simulink model "HumanoidModel_ResidualRL"  (R2025b)
settings: Solver=daessc  StartTime=0.0  StopTime=11  RelTol=1e-3  AbsTol=1e-3
PreLoadFcn:
  | addpath(fullfile('ImportedURDFSupport','Geometries'));
  | addpath(fullfile('ImportedURDFSupport','Data'));
undefined symbols (not defined in the file): kd_ankle_vy, kd_ankle_wx, kd_hip_sag_vx, kd_hip_sag_wy, kd_hip_vy, kd_hip_vz, kd_hip_wx, kp_ankle_qx, kp_ankle_y, kp_hip_dz, kp_hip_qx, kp_hip_sag_qy, kp_hip_sag_x, kp_hip_y, params, residualRLActionPenaltyWeight, residualRLActionRatePenaltyWeight, residualRLAliveReward, residualRLChannelMap, residualRLEnabled, residualRLLeftFootLoadMap, residualRLManualAction, residualRLNominalFootLoad_N, residualRLObservationInverseScales, residualRLRewardStateWeights, residualRLRightFootLoadMap, residualRLSampleTime_s, residualRLTerminalPenalty, residualRLTorqueLimit_Nm, residualRLUseAgent, robustnessForceDuration_s, robustnessForceStart_s, robustnessForceVector_N, Rx_ref, u_ankle_pitch, u_hip_frontal, u_hip_sagittal, u_knee, u_shoulder_frontal, X, Y, y_ref, Z
libraries: sm_lib x155, nesl_utility x96, simulink_extras x18, simulink x5, robotmaniplib x1, rllib x1
(part 2 of 6)

== system HumanoidModel_ResidualRL/Torque Reordering1 ==
  In1 : Inport
  Bus Creator3 : BusCreator  Inputs=12
  Demux : Demux  Outputs=22
  Gain{1..12} (12 alike) : Gain
  Scope5 : Scope
      settings: ActiveDisplayYMinimum=-30.863133772002811  ActiveDisplayYMaximum=8.6957298127878211  DataLoggingVariableName=ScopeData5
  Out1 : Outport
  wires:
  In1/1 -> Demux/1
  Bus Creator3/1 -> Scope5/1, Out1/1
  Demux/12 -> Gain12/1  "right_hip_frontal"
  Demux/14 -> Gain6/1  "right_knee"
  Demux/16 -> Gain11/1  "right_ankle_pitch"
  Demux/13 -> Gain8/1  "right_hip_sagittal"
  Demux/11 -> Gain7/1  "right_hip_transverse"
  Demux/15 -> Gain10/1  "right_ankle_roll"
  Demux/18 -> Gain4/1  "left_hip_frontal"
  Gain4/1 -> Bus Creator3/7  "left_hip_frontal"
  Demux/20 -> Gain1/1  "left_knee"
  Gain1/1 -> Bus Creator3/8  "left_knee"
  Demux/22 -> Gain9/1  "left_ankle_pitch"
  Demux/19 -> Gain2/1  "left_hip_sagittal"
  Gain2/1 -> Bus Creator3/10  "left_hip_sagittal"
  Demux/17 -> Gain3/1  "left_hip_transverse"
  Gain3/1 -> Bus Creator3/11  "left_hip_transverse"
  Demux/21 -> Gain5/1  "left_ankle_roll"
  Gain5/1 -> Bus Creator3/12  "left_ankle_roll"
  Gain6/1 -> Bus Creator3/2  "right_knee"
  Gain7/1 -> Bus Creator3/5  "right_hip_transverse"
  Gain8/1 -> Bus Creator3/4  "right_hip_sagittal"
  Gain9/1 -> Bus Creator3/9  "left_ankle_pitch"
  Gain10/1 -> Bus Creator3/6  "right_ankle_roll"
  Gain11/1 -> Bus Creator3/3  "right_ankle_pitch"
  Gain12/1 -> Bus Creator3/1  "right_hip_frontal"

== system HumanoidModel_ResidualRL/Control Input/Left ankle feedback ==
  qx : Inport
  wx : Inport  Port=2
  vy : Inport  Port=3
  y : Inport  Port=4
  Constant2 : Constant  Value=u_ankle_pitch
  Gain : Gain  Gain=kd_ankle_wx
  Gain1 : Gain  Gain=kp_ankle_qx
  Gain2 : Gain  Gain=kp_ankle_y
  Gain3 : Gain  Gain=kd_ankle_vy
  Subtract : Sum  Inputs=+-
  Subtract1 : Sum  Inputs=+-
  Sum : Sum  Inputs=|++++
  Sum1 : Sum  Inputs=|++
  qx_ref : Constant  Value=Rx_ref
  y_ref : Constant  Value=y_ref
  Out1 : Outport
  wires:
  Sum/1 -> Out1/1
  Subtract/1 -> Gain1/1
  Gain1/1 -> Sum/1
  Gain/1 -> Sum/2
  wx/1 -> Gain/1
  qx/1 -> Subtract/1
  qx_ref/1 -> Subtract/2
  Sum1/1 -> Sum/4
  Gain3/1 -> Sum1/2
  y_ref/1 -> Subtract1/2
  Gain2/1 -> Sum1/1
  Subtract1/1 -> Gain2/1
  y/1 -> Subtract1/1
  vy/1 -> Gain3/1
  Constant2/1 -> Sum/3

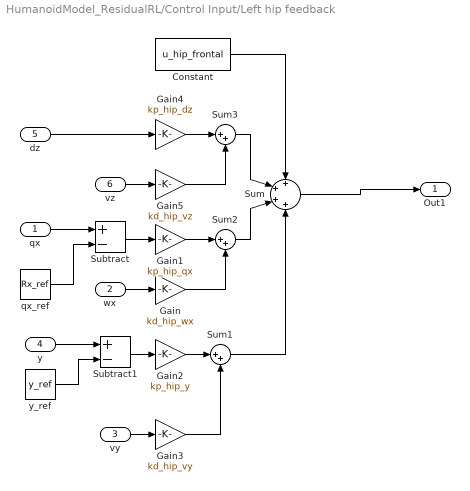
== system HumanoidModel_ResidualRL/Control Input/Left hip feedback ==
  qx : Inport
  wx : Inport  Port=2
  vy : Inport  Port=3
  y : Inport  Port=4
  dz : Inport  Port=5
  vz : Inport  Port=6
  Constant : Constant  Value=u_hip_frontal
  Gain : Gain  Gain=kd_hip_wx
  Gain1 : Gain  Gain=kp_hip_qx
  Gain2 : Gain  Gain=kp_hip_y
  Gain3 : Gain  Gain=kd_hip_vy
  Gain4 : Gain  Gain=kp_hip_dz
  Gain5 : Gain  Gain=kd_hip_vz
  Subtract : Sum  Inputs=+-
  Subtract1 : Sum  Inputs=+-
  Sum : Sum  Inputs=++++
  Sum1 : Sum  Inputs=|++
  Sum2 : Sum  Inputs=|++
  Sum3 : Sum  Inputs=|++
  qx_ref : Constant  Value=Rx_ref
  y_ref : Constant  Value=y_ref
  Out1 : Outport
  wires:
  Gain1/1 -> Sum2/1
  Gain4/1 -> Sum3/1
  Sum3/1 -> Sum/2
  vz/1 -> Gain5/1
  Gain2/1 -> Sum1/1
  Gain/1 -> Sum2/2
  Subtract1/1 -> Gain2/1
  Sum1/1 -> Sum/4
  Subtract/1 -> Gain1/1
  wx/1 -> Gain/1
  Gain3/1 -> Sum1/2
  y/1 -> Subtract1/1
  vy/1 -> Gain3/1
  qx/1 -> Subtract/1
  y_ref/1 -> Subtract1/2
  Sum/1 -> Out1/1
  Gain5/1 -> Sum3/2
  Sum2/1 -> Sum/3
  qx_ref/1 -> Subtract/2
  dz/1 -> Gain4/1
  Constant/1 -> Sum/1

== system HumanoidModel_ResidualRL/Control Input/Left hip sagittal feedback ==
  qy : Inport
  wy : Inport  Port=2
  x : Inport  Port=3
  vx : Inport  Port=4
  Gain : Gain  Gain=kp_hip_sag_qy
  Gain1 : Gain  Gain=kd_hip_sag_wy
  Gain2 : Gain  Gain=kd_hip_sag_vx
  Gain3 : Gain  Gain=kp_hip_sag_x
  Nominal hip sagittal u : Constant  Value=u_hip_sagittal
  Sum : Sum  Inputs=+++++
  Out1 : Outport
  wires:
  Sum/1 -> Out1/1
  vx/1 -> Gain2/1
  x/1 -> Gain3/1
  Gain2/1 -> Sum/4
  Gain3/1 -> Sum/3
  Gain1/1 -> Sum/2
  Gain/1 -> Sum/1
  wy/1 -> Gain1/1
  qy/1 -> Gain/1
  Nominal hip sagittal u/1 -> Sum/5

== system HumanoidModel_ResidualRL/Control Input/Right ankle feedback ==
  qx : Inport
  wx : Inport  Port=2
  vy : Inport  Port=3
  y : Inport  Port=4
  Constant2 : Constant  Value=u_ankle_pitch
  Gain : Gain  Gain=kd_ankle_wx
  Gain1 : Gain  Gain=kp_ankle_qx
  Gain2 : Gain  Gain=kp_ankle_y
  Gain3 : Gain  Gain=kd_ankle_vy
  Subtract : Sum  Inputs=+-
  Subtract1 : Sum  Inputs=+-
  Sum : Sum  Inputs=|++++
  Sum1 : Sum  Inputs=|++
  qx_ref : Constant  Value=Rx_ref
  y_ref : Constant  Value=y_ref
  Out1 : Outport
  wires:
  wx/1 -> Gain/1
  Gain/1 -> Sum/2
  Gain1/1 -> Sum/1
  Sum/1 -> Out1/1
  Subtract/1 -> Gain1/1
  qx/1 -> Subtract/1
  qx_ref/1 -> Subtract/2
  Sum1/1 -> Sum/4
  Gain3/1 -> Sum1/2
  y_ref/1 -> Subtract1/2
  Gain2/1 -> Sum1/1
  Subtract1/1 -> Gain2/1
  y/1 -> Subtract1/1
  vy/1 -> Gain3/1
  Constant2/1 -> Sum/3

== system HumanoidModel_ResidualRL/Control Input/Right hip feedback ==
  qx : Inport
  wx : Inport  Port=2
  vy : Inport  Port=3
  y : Inport  Port=4
  dz : Inport  Port=5
  vz : Inport  Port=6
  Constant : Constant  Value=u_hip_frontal
  Gain : Gain  Gain=kd_hip_wx
  Gain1 : Gain  Gain=kp_hip_qx
  Gain2 : Gain  Gain=kp_hip_y
  Gain3 : Gain  Gain=kd_hip_vy
  Gain4 : Gain  Gain=kp_hip_dz
  Gain5 : Gain  Gain=kd_hip_vz
  Subtract : Sum  Inputs=+-
  Subtract1 : Sum  Inputs=+-
  Sum : Sum  Inputs=++++
  Sum1 : Sum  Inputs=|++
  Sum2 : Sum  Inputs=|++
  Sum3 : Sum  Inputs=|++
  qx_ref : Constant  Value=Rx_ref
  y_ref : Constant  Value=y_ref
  Out1 : Outport
  wires:
  qx_ref/1 -> Subtract/2
  qx/1 -> Subtract/1
  Subtract/1 -> Gain1/1
  Sum/1 -> Out1/1
  wx/1 -> Gain/1
  y/1 -> Subtract1/1
  y_ref/1 -> Subtract1/2
  Subtract1/1 -> Gain2/1
  Gain2/1 -> Sum1/1
  vy/1 -> Gain3/1
  Gain3/1 -> Sum1/2
  Sum1/1 -> Sum/4
  Gain1/1 -> Sum2/1
  Gain/1 -> Sum2/2
  Sum2/1 -> Sum/3
  dz/1 -> Gain4/1
  vz/1 -> Gain5/1
  Gain4/1 -> Sum3/1
  Gain5/1 -> Sum3/2
  Sum3/1 -> Sum/2
  Constant/1 -> Sum/1  "Right Hip Frontal"

== system HumanoidModel_ResidualRL/Control Input/Right hip sagittal feedback ==
  qy : Inport
  wy : Inport  Port=2
  x : Inport  Port=3
  vx : Inport  Port=4
  Gain : Gain  Gain=kp_hip_sag_qy
  Gain1 : Gain  Gain=kd_hip_sag_wy
  Gain2 : Gain  Gain=kd_hip_sag_vx
  Gain3 : Gain  Gain=kp_hip_sag_x
  Nominal hip sagittal u : Constant  Value=u_hip_sagittal
  Sum : Sum  Inputs=+++++
  Out1 : Outport
  wires:
  qy/1 -> Gain/1
  wy/1 -> Gain1/1
  Gain/1 -> Sum/1
  Gain1/1 -> Sum/2
  Gain3/1 -> Sum/3
  Gain2/1 -> Sum/4
  x/1 -> Gain3/1
  vx/1 -> Gain2/1
  Sum/1 -> Out1/1
  Nominal hip sagittal u/1 -> Sum/5

== system HumanoidModel_ResidualRL/Humanoid Robot/Arms ==
  Torque Input : Inport
  Bus Creator : BusCreator  Inputs=2
  Demux : Demux  Outputs=2
  Left Arm : Subsystem
  Right Arm : Subsystem
  Right Shoulder : PMIOPort  Side=Left
  Left Shoulder : PMIOPort  Port=2  Side=Left
  Arms Joint Sensing : Outport
  wires:
  Torque Input/1 -> Demux/1
  Demux/1 -> Right Arm/1(Torque Input)
  Demux/2 -> Left Arm/1(Torque Input)
  Bus Creator/1 -> Arms Joint Sensing/1
  Left Arm/1(Sensing) -> Bus Creator/2
  Right Arm/1(Sensing) -> Bus Creator/1
  connections:
  Left Arm/LConn1 -- Left Shoulder/RConn1
  Right Arm/LConn1 -- Right Shoulder/RConn1

== system HumanoidModel_ResidualRL/Humanoid Robot/Foot Contact Modelling ==
  Bus Creator : BusCreator  Inputs=2
  Bus Creator1 : BusCreator  Inputs=2
  Left Foot Contact : Subsystem  AncestorBlock=sm_humanoid_walker_lib/Humanoid Robot/Foot Contact Modelling/Right Foot Contact
  Right Foot Contact : Subsystem
  Right Foot Contact Points : PMIOPort  Side=Left
  Left Foot Contact Points : PMIOPort  Port=2  Side=Left
  Feet Contact : PMIOPort  Port=3  Side=Left
  Total Contact Sensing : Outport
  Contact Sensing : Outport  Port=2
  wires:
  Bus Creator/1 -> Total Contact Sensing/1
  Right Foot Contact/1(Foot Force) -> Bus Creator/1  "rightContactTotal"
  Left Foot Contact/1(Foot Force) -> Bus Creator/2  "leftContactTotal"
  Bus Creator1/1 -> Contact Sensing/1
  Right Foot Contact/2(Contact Point Forces) -> Bus Creator1/1  "rightContact"
  Left Foot Contact/2(Contact Point Forces) -> Bus Creator1/2  "leftContact"
  connections:
  Left Foot Contact/LConn1 -- Left Foot Contact Points/RConn1
  Feet Contact/RConn1 -- Left Foot Contact/RConn1 -- Right Foot Contact/RConn1
  Right Foot Contact/LConn1 -- Right Foot Contact Points/RConn1

== system HumanoidModel_ResidualRL/Humanoid Robot/Legs ==
  Torque Input : Inport
  Bus Creator : BusCreator  Inputs=2
  Demux : Demux  Outputs=2
  Left Leg : Subsystem
  Right leg : Subsystem
  Right Hip : PMIOPort  Side=Left
  Right Foot : PMIOPort  Port=2  Side=Right
  Left Foot : PMIOPort  Port=3  Side=Right
  Left Hip : PMIOPort  Port=4  Side=Left
  Joint Sensing : Outport
  wires:
  Demux/2 -> Left Leg/1(Torque Input)
  Left Leg/1(Sensing) -> Bus Creator/2
  Torque Input/1 -> Demux/1
  Demux/1 -> Right leg/1(Torque Input)
  Bus Creator/1 -> Joint Sensing/1
  Right leg/1(Sensing) -> Bus Creator/1
  connections:
  Right Hip/RConn1 -- Right leg/LConn1
  Left Foot/RConn1 -- Left Leg/RConn1
  Right Foot/RConn1 -- Right leg/RConn1
  Left Hip/RConn1 -- Left Leg/LConn1

== system HumanoidModel_ResidualRL/Humanoid Robot/Torso and Head ==
  Cover : sm_lib/Body Elements/File Solid  ExtGeomFileName=sm_humanoid_walker_cover.stp  UnitType=FromFile  ExtGeomFileUnits=m  StepReaderType=HEX  ExportConvexHullGeometry=off  InertiaType=CalculateFromGeometry  BasedOnType=Density  Density=headDensity  DensityUnits=kg/m^3  Mass=0  MassUnits=kg  CenterOfMass=[0, 0, 0]  CenterOfMassUnits=m  MomentsOfInertia=[0, 0, 0]  MomentsOfInertiaUnits=kg*m^2  ProductsOfInertia=[0, 0, 0]  ProductsOfInertiaUnits=kg*m^2  GraphicType=FromGeometry  MarkerShape=Sphere  MarkerSize=10  GraphicVisPropType=SimpleVisualProperties  GraphicDiffuseColor=[1, 1, 1]  GraphicOpacity=1  GraphicSpecularColor=[0.5 0.5 0.5 1.0]  GraphicAmbientColor=[0.15 0.15 0.15 1.0]  GraphicEmissiveColor=[0.0 0.0 0.0 1.0]  GraphicShininess=75  DoExposeReferenceFrame=on  SerializedFrames=<Frames/>
  Head : sm_lib/Body Elements/File Solid  ExtGeomFileName=sm_humanoid_walker_head.stp  UnitType=FromFile  ExtGeomFileUnits=m  StepReaderType=HEX  ExportConvexHullGeometry=off  InertiaType=CalculateFromGeometry  BasedOnType=Density  Density=headDensity  DensityUnits=kg/m^3  Mass=0  MassUnits=kg  CenterOfMass=[0, 0, 0]  CenterOfMassUnits=m  MomentsOfInertia=[0, 0, 0]  MomentsOfInertiaUnits=kg*m^2  ProductsOfInertia=[0, 0, 0]  ProductsOfInertiaUnits=kg*m^2  GraphicType=FromGeometry  MarkerShape=Sphere  MarkerSize=10  GraphicVisPropType=SimpleVisualProperties  GraphicDiffuseColor=[0.0 0.0 0.0]  GraphicOpacity=1  GraphicSpecularColor=[0.5 0.5 0.5 1.0]  GraphicAmbientColor=[0.15 0.15 0.15 1.0]  GraphicEmissiveColor=[0.0 0.0 0.0 1.0]  GraphicShininess=75  DoExposeReferenceFrame=on  SerializedFrames=<Frames/>
  Head Origin Transformation : sm_lib/Frames and Transforms/Rigid Transform  RotationMethod=RotationSequence  FollAlignAxisA=+X  BaseAlignAxisA=+Y  FollAlignAxisB=+Y  BaseAlignAxisB=+Z  RotationStandardAxis=+Z  RotationAngle=0.0  RotationAngleUnits=deg  RotationArbitraryAxis=[0 0 1]  RotationSequenceAxes=BaseAxes  RotationSequence=XYZ  RotationSequenceAngles=[0, 0, 0]  RotationSequenceAnglesUnits=rad  RotationMatrix=[1 0 0; 0 1 0; 0 0 1]  Quaternion=[1 0 0 0]  TranslationMethod=Cartesian  TranslationCartesianOffset=[0, 0, 0.06414]*3.5  TranslationCartesianOffsetUnits=m  TranslationStandardAxis=+Z  TranslationStandardOffset=0  TranslationStandardOffsetUnits=m  TranslationROffset=0  TranslationROffsetUnits=m  TranslationThetaOffset=0  TranslationThetaOffsetUnits=deg  TranslationZOffset=0  TranslationZOffsetUnits=m
  Neck : sm_lib/Body Elements/File Solid  ExtGeomFileName=sm_humanoid_walker_neck.stp  UnitType=FromFile  ExtGeomFileUnits=m  StepReaderType=HEX  ExportConvexHullGeometry=off  InertiaType=CalculateFromGeometry  BasedOnType=Density  Density=headDensity  DensityUnits=kg/m^3  Mass=0  MassUnits=kg  CenterOfMass=[0, 0, 0]  CenterOfMassUnits=m  MomentsOfInertia=[0, 0, 0]  MomentsOfInertiaUnits=kg*m^2  ProductsOfInertia=[0, 0, 0]  ProductsOfInertiaUnits=kg*m^2  GraphicType=FromGeometry  MarkerShape=Sphere  MarkerSize=10  GraphicVisPropType=SimpleVisualProperties  GraphicDiffuseColor=[0.0 0.0 0.0]  GraphicOpacity=1  GraphicSpecularColor=[0.5 0.5 0.5 1.0]  GraphicAmbientColor=[0.15 0.15 0.15 1.0]  GraphicEmissiveColor=[0.0 0.0 0.0 1.0]  GraphicShininess=75  DoExposeReferenceFrame=on  SerializedFrames=<Frames/>
  Neck Origin Tranformation : sm_lib/Frames and Transforms/Rigid Transform  RotationMethod=RotationSequence  FollAlignAxisA=+X  BaseAlignAxisA=+Y  FollAlignAxisB=+Y  BaseAlignAxisB=+Z  RotationStandardAxis=+Z  RotationAngle=0.0  RotationAngleUnits=deg  RotationArbitraryAxis=[0 0 1]  RotationSequenceAxes=BaseAxes  RotationSequence=XYZ  RotationSequenceAngles=[0, 0, 0]  RotationSequenceAnglesUnits=rad  RotationMatrix=[1 0 0; 0 1 0; 0 0 1]  Quaternion=[1 0 0 0]  TranslationMethod=Cartesian  TranslationCartesianOffset=[0, 0, 0.01016]*3.5  TranslationCartesianOffsetUnits=m  TranslationStandardAxis=+Z  TranslationStandardOffset=0  TranslationStandardOffsetUnits=m  TranslationROffset=0  TranslationROffsetUnits=m  TranslationThetaOffset=0  TranslationThetaOffsetUnits=deg  TranslationZOffset=0  TranslationZOffsetUnits=m
  Shoulder : sm_lib/Body Elements/File Solid  ExtGeomFileName=sm_humanoid_walker_shoulder.stp  UnitType=FromFile  ExtGeomFileUnits=m  StepReaderType=HEX  ExportConvexHullGeometry=off  InertiaType=CalculateFromGeometry  BasedOnType=Density  Density=shoulderDensity  DensityUnits=kg/m^3  Mass=0  MassUnits=kg  CenterOfMass=[0, 0, 0]  CenterOfMassUnits=m  MomentsOfInertia=[0, 0, 0]  MomentsOfInertiaUnits=kg*m^2  ProductsOfInertia=[0, 0, 0]  ProductsOfInertiaUnits=kg*m^2  GraphicType=FromGeometry  MarkerShape=Sphere  MarkerSize=10  GraphicVisPropType=SimpleVisualProperties  GraphicDiffuseColor=[1.0 0.6 0.6]  GraphicOpacity=1  GraphicSpecularColor=[0.5 0.5 0.5 1.0]  GraphicAmbientColor=[0.15 0.15 0.15 1.0]  GraphicEmissiveColor=[0.0 0.0 0.0 1.0]  GraphicShininess=75  DoExposeReferenceFrame=on  SerializedFrames=<Frames/>
  Shoulder Origin Transformation : sm_lib/Frames and Transforms/Rigid Transform  RotationMethod=RotationSequence  FollAlignAxisA=+X  BaseAlignAxisA=+Y  FollAlignAxisB=+Y  BaseAlignAxisB=+Z  RotationStandardAxis=+Z  RotationAngle=0.0  RotationAngleUnits=deg  RotationArbitraryAxis=[0 0 1]  RotationSequenceAxes=BaseAxes  RotationSequence=XYZ  RotationSequenceAngles=[0, 0, 0]  RotationSequenceAnglesUnits=rad  RotationMatrix=[1 0 0; 0 1 0; 0 0 1]  Quaternion=[1 0 0 0]  TranslationMethod=Cartesian  TranslationCartesianOffset=[0, 0, -0.0399]*3.5  TranslationCartesianOffsetUnits=m  TranslationStandardAxis=+Z  TranslationStandardOffset=0  TranslationStandardOffsetUnits=m  TranslationROffset=0  TranslationROffsetUnits=m  TranslationThetaOffset=0  TranslationThetaOffsetUnits=deg  TranslationZOffset=0  TranslationZOffsetUnits=m
  Trunk : sm_lib/Body Elements/File Solid  ExtGeomFileName=sm_humanoid_walker_trunk.stp  UnitType=FromFile  ExtGeomFileUnits=km  StepReaderType=HEX  ExportConvexHullGeometry=off  InertiaType=CalculateFromGeometry  BasedOnType=Density  Density=trunkDensity  DensityUnits=kg/m^3  Mass=0  MassUnits=kg  CenterOfMass=[0, 0, 0]  CenterOfMassUnits=m  MomentsOfInertia=[0, 0, 0]  MomentsOfInertiaUnits=kg*m^2  ProductsOfInertia=[0, 0, 0]  ProductsOfInertiaUnits=kg*m^2  GraphicType=FromGeometry  MarkerShape=Sphere  MarkerSize=10  GraphicVisPropType=SimpleVisualProperties  GraphicDiffuseColor=[1.0 0.2 0.2]  GraphicOpacity=1  GraphicSpecularColor=[0.5 0.5 0.5 1.0]  GraphicAmbientColor=[0.15 0.15 0.15 1.0]  GraphicEmissiveColor=[0.0 0.0 0.0 1.0]  GraphicShininess=75  DoExposeReferenceFrame=on  SerializedFrames=<Frames/>
  Torso : PMIOPort  Side=Left
  Torso Ref : PMIOPort  Port=2  Side=Right
  connections:
  Neck/RConn1 -- Head Origin Transformation/LConn1 -- Neck Origin Tranformation/RConn1
  Neck Origin Tranformation/LConn1 -- Shoulder Origin Transformation/RConn1 -- Shoulder/RConn1
  Cover/RConn1 -- Head Origin Transformation/RConn1 -- Head/RConn1
  Trunk/RConn1 -- Torso/RConn1 -- Torso Ref/RConn1 -- Shoulder Origin Transformation/LConn1

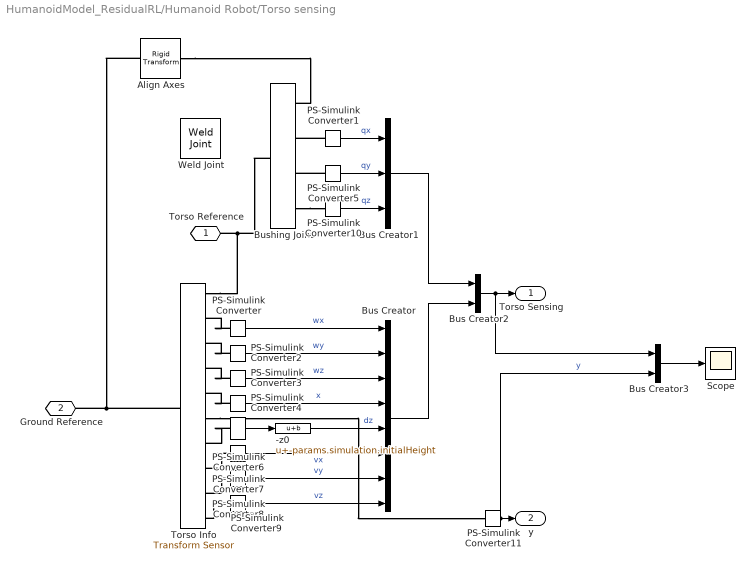
== system HumanoidModel_ResidualRL/Humanoid Robot/Torso sensing ==
  -z0 : Bias  Bias=-params.simulation.initialHeight  SaturateOnIntegerOverflow=off
  Align Axes : sm_lib/Frames and Transforms/Rigid Transform  RotationMethod=StandardAxis  FollAlignAxisA=+X  BaseAlignAxisA=+Y  FollAlignAxisB=+Y  BaseAlignAxisB=+Z  RotationStandardAxis=+Z  RotationAngle=180  RotationAngleUnits=deg  RotationArbitraryAxis=[0 0 1]  RotationSequenceAxes=FollowerAxes  RotationSequence=XYX  RotationSequenceAngles=[0 0 0]  RotationSequenceAnglesUnits=deg  RotationMatrix=[1 0 0; 0 1 0; 0 0 1]  Quaternion=[1 0 0 0]  TranslationMethod=None  TranslationCartesianOffset=[0 0 0]  TranslationCartesianOffsetUnits=m  TranslationStandardAxis=+Z  TranslationStandardOffset=0  TranslationStandardOffsetUnits=m  TranslationROffset=0  TranslationROffsetUnits=m  TranslationThetaOffset=0  TranslationThetaOffsetUnits=deg  TranslationZOffset=0  TranslationZOffsetUnits=m
  Bus Creator : BusCreator  Inputs=8
  Bus Creator1 : BusCreator  Inputs=3
  Bus Creator2 : BusCreator  Inputs=2
  Bus Creator3 : BusCreator  Inputs=2
  Bushing Joint : sm_lib/Joints/Bushing Joint  JointMode=Normal  CompositeWrenchDir=FollowerOnBase  CompositeWrenchFrame=BaseFrame  SenseConstraintForce=off  SenseConstraintTorque=off  SenseTotalForce=off  SenseTotalTorque=off  PxPositionTargetSpecify=off  PxPositionTargetPriority=High  PxPositionTargetValue=0  PxPositionTargetValueUnits=m  PxVelocityTargetSpecify=off  PxVelocityTargetPriority=High  PxVelocityTargetValue=0  PxVelocityTargetValueUnits=m/s  PxEquilibriumPosition=0  PxEquilibriumPositionUnits=m  PxSpringStiffness=0  PxSpringStiffnessUnits=N/m  PxDampingCoefficient=0  PxDampingCoefficientUnits=N/(m/s)  PxLowerLimitSpecify=off  PxLowerLimitBound=-0.02  PxLowerLimitBoundUnits=m  PxLowerLimitStiffness=1e6  PxLowerLimitStiffnessUnits=N/m  PxLowerLimitDamping=1e3  PxLowerLimitDampingUnits=N/(m/s)  PxLowerLimitTransitionRegionWidth=1e-4  PxLowerLimitTransitionRegionWidthUnits=m  PxUpperLimitSpecify=off  PxUpperLimitBound=0.02  PxUpperLimitBoundUnits=m  PxUpperLimitStiffness=1e6  PxUpperLimitStiffnessUnits=N/m  PxUpperLimitDamping=1e3  PxUpperLimitDampingUnits=N/(m/s)  PxUpperLimitTransitionRegionWidth=1e-4  PxUpperLimitTransitionRegionWidthUnits=m  PxTorqueActuationMode=NoTorque  PxMotionActuationMode=ComputedMotion  PxSensePosition=off  PxSenseVelocity=off  PxSenseAcceleration=off  PxSenseTorqueForce=off  PxSenseLowerLimitTorqueForce=off  PxSenseUpperLimitTorqueForce=off  PyPositionTargetSpecify=off  PyPositionTargetPriority=High  PyPositionTargetValue=0  PyPositionTargetValueUnits=m  PyVelocityTargetSpecify=off  PyVelocityTargetPriority=High  PyVelocityTargetValue=0  PyVelocityTargetValueUnits=m/s  PyEquilibriumPosition=0  PyEquilibriumPositionUnits=m  PySpringStiffness=0  PySpringStiffnessUnits=N/m  PyDampingCoefficient=0  PyDampingCoefficientUnits=N/(m/s)  PyLowerLimitSpecify=off  PyLowerLimitBound=-1  PyLowerLimitBoundUnits=m  PyLowerLimitStiffness=1e6  PyLowerLimitStiffnessUnits=N/m  PyLowerLimitDamping=1e3  PyLowerLimitDampingUnits=N/(m/s)  PyLowerLimitTransitionRegionWidth=1e-4  PyLowerLimitTransitionRegionWidthUnits=m  PyUpperLimitSpecify=off  PyUpperLimitBound=1  PyUpperLimitBoundUnits=m  PyUpperLimitStiffness=1e6  PyUpperLimitStiffnessUnits=N/m  PyUpperLimitDamping=1e3  PyUpperLimitDampingUnits=N/(m/s)  PyUpperLimitTransitionRegionWidth=1e-4  PyUpperLimitTransitionRegionWidthUnits=m  PyTorqueActuationMode=NoTorque  PyMotionActuationMode=ComputedMotion  PySensePosition=off  PySenseVelocity=off  PySenseAcceleration=off  PySenseTorqueForce=off  PySenseLowerLimitTorqueForce=off  PySenseUpperLimitTorqueForce=off  PzPositionTargetSpecify=on  PzPositionTargetPriority=High  PzPositionTargetValue=-params.simulation.initialHeight  PzPositionTargetValueUnits=m  PzVelocityTargetSpecify=off  PzVelocityTargetPriority=High  PzVelocityTargetValue=0  PzVelocityTargetValueUnits=m/s  PzEquilibriumPosition=0  PzEquilibriumPositionUnits=m  PzSpringStiffness=0  PzSpringStiffnessUnits=N/m  PzDampingCoefficient=params.simulation.worldDamping  PzDampingCoefficientUnits=N/(m/s)  PzLowerLimitSpecify=off  PzLowerLimitBound=-1  PzLowerLimitBoundUnits=m  PzLowerLimitStiffness=1e6  PzLowerLimitStiffnessUnits=N/m  PzLowerLimitDamping=1e3  PzLowerLimitDampingUnits=N/(m/s)  PzLowerLimitTransitionRegionWidth=1e-4  PzLowerLimitTransitionRegionWidthUnits=m  PzUpperLimitSpecify=off  PzUpperLimitBound=1  PzUpperLimitBoundUnits=m  PzUpperLimitStiffness=1e6  PzUpperLimitStiffnessUnits=N/m  PzUpperLimitDamping=1e3  PzUpperLimitDampingUnits=N/(m/s)  PzUpperLimitTransitionRegionWidth=1e-4  PzUpperLimitTransitionRegionWidthUnits=m  PzTorqueActuationMode=NoTorque  PzMotionActuationMode=ComputedMotion  PzSensePosition=off  PzSenseVelocity=off  PzSenseAcceleration=off  PzSenseTorqueForce=off  PzSenseLowerLimitTorqueForce=off  PzSenseUpperLimitTorqueForce=off  RxPositionTargetSpecify=on  RxPositionTargetPriority=High  RxPositionTargetValue=-10  RxPositionTargetValueUnits=deg  RxVelocityTargetSpecify=off  RxVelocityTargetPriority=High  RxVelocityTargetValue=0  RxVelocityTargetValueUnits=deg/s  RxEquilibriumPosition=0  RxEquilibriumPositionUnits=deg  RxSpringStiffness=0  RxSpringStiffnessUnits=N*m/deg  RxDampingCoefficient=params.simulation.worldDamping  RxDampingCoefficientUnits=N*m/(deg/s)  RxLowerLimitSpecify=off  RxLowerLimitBound=-90  RxLowerLimitBoundUnits=deg  RxLowerLimitStiffness=1e4  RxLowerLimitStiffnessUnits=N*m/deg  RxLowerLimitDamping=10  RxLowerLimitDampingUnits=N*m/(deg/s)  RxLowerLimitTransitionRegionWidth=0.1  RxLowerLimitTransitionRegionWidthUnits=deg  RxUpperLimitSpecify=off  RxUpperLimitBound=90  RxUpperLimitBoundUnits=deg  RxUpperLimitStiffness=1e4  RxUpperLimitStiffnessUnits=N*m/deg  RxUpperLimitDamping=10  RxUpperLimitDampingUnits=N*m/(deg/s)  RxUpperLimitTransitionRegionWidth=0.1  RxUpperLimitTransitionRegionWidthUnits=deg  RxTorqueActuationMode=NoTorque  RxMotionActuationMode=ComputedMotion  RxSensePosition=on  RxSenseVelocity=off  RxSenseAcceleration=off  RxSenseTorqueForce=off  RxSenseLowerLimitTorqueForce=off  RxSenseUpperLimitTorqueForce=off  RyPositionTargetSpecify=off  RyPositionTargetPriority=High  RyPositionTargetValue=0  RyPositionTargetValueUnits=deg  RyVelocityTargetSpecify=off  RyVelocityTargetPriority=High  RyVelocityTargetValue=0  RyVelocityTargetValueUnits=deg/s  RyEquilibriumPosition=0  RyEquilibriumPositionUnits=deg  RySpringStiffness=0  RySpringStiffnessUnits=N*m/deg  RyDampingCoefficient=params.simulation.worldDamping  RyDampingCoefficientUnits=N*m/(deg/s)  RyLowerLimitSpecify=off  RyLowerLimitBound=-90  RyLowerLimitBoundUnits=deg  RyLowerLimitStiffness=1e4  RyLowerLimitStiffnessUnits=N*m/deg  RyLowerLimitDamping=10  RyLowerLimitDampingUnits=N*m/(deg/s)  RyLowerLimitTransitionRegionWidth=0.1  RyLowerLimitTransitionRegionWidthUnits=deg  RyUpperLimitSpecify=off  RyUpperLimitBound=90  RyUpperLimitBoundUnits=deg  RyUpperLimitStiffness=1e4  RyUpperLimitStiffnessUnits=N*m/deg  RyUpperLimitDamping=10  RyUpperLimitDampingUnits=N*m/(deg/s)  RyUpperLimitTransitionRegionWidth=0.1  RyUpperLimitTransitionRegionWidthUnits=deg  RyTorqueActuationMode=NoTorque  RyMotionActuationMode=ComputedMotion  RySensePosition=on  RySenseVelocity=off  RySenseAcceleration=off  RySenseTorqueForce=off  RySenseLowerLimitTorqueForce=off  RySenseUpperLimitTorqueForce=off  RzPositionTargetSpecify=on  RzPositionTargetPriority=High  RzPositionTargetValue=0  RzPositionTargetValueUnits=deg  RzVelocityTargetSpecify=off  RzVelocityTargetPriority=High  RzVelocityTargetValue=0  RzVelocityTargetValueUnits=deg/s  RzEquilibriumPosition=0  RzEquilibriumPositionUnits=deg  RzSpringStiffness=0  RzSpringStiffnessUnits=N*m/deg  RzDampingCoefficient=params.simulation.worldDamping  RzDampingCoefficientUnits=N*m/(deg/s)  RzLowerLimitSpecify=off  RzLowerLimitBound=-90  RzLowerLimitBoundUnits=deg  RzLowerLimitStiffness=1e4  RzLowerLimitStiffnessUnits=N*m/deg  RzLowerLimitDamping=10  RzLowerLimitDampingUnits=N*m/(deg/s)  RzLowerLimitTransitionRegionWidth=0.1  RzLowerLimitTransitionRegionWidthUnits=deg  RzUpperLimitSpecify=off  RzUpperLimitBound=90  RzUpperLimitBoundUnits=deg  RzUpperLimitStiffness=1e4  RzUpperLimitStiffnessUnits=N*m/deg  RzUpperLimitDamping=10  RzUpperLimitDampingUnits=N*m/(deg/s)  RzUpperLimitTransitionRegionWidth=0.1  RzUpperLimitTransitionRegionWidthUnits=deg  RzTorqueActuationMode=NoTorque  RzMotionActuationMode=ComputedMotion  RzSensePosition=on  RzSenseVelocity=off  RzSenseAcceleration=off  RzSenseTorqueForce=off  RzSenseLowerLimitTorqueForce=off  RzSenseUpperLimitTorqueForce=off
  PS-Simulink Converter{,1..11} (12 alike) : nesl_utility/PS-Simulink Converter  PhysicalDomain=network_engine_domain  SubClassName=ps_output  LeftPortType=input  RightPortType=output  PseudoPeriodic=off  Frequencies=[]  VectorFormat=1-D array  Unit=inherit  AffineConversion=off
  Scope : Scope
      settings: ActiveDisplayYMinimum=-1.8812137497158752  ActiveDisplayYMaximum=2.378403432232306
  Torso Info : sm_lib/Frames and Transforms/Transform Sensor  MeasurementFrame=World  RotationSequence=XYX  SenseAngle=off  SenseAxis=off  SenseQ=off  SenseR=off  SenseRotationSequence=off  SenseOmegaX=on  SenseOmegaY=on  SenseOmegaZ=on  SenseOmega=off  SenseQDot=off  SenseRDot=off  SenseRotationSequenceDot=off  SenseAlphaX=off  SenseAlphaY=off  SenseAlphaZ=off  SenseAlpha=off  SenseQDDot=off  SenseRDDot=off  SenseX=on  SenseY=on  SenseZ=on  SenseXYZ=off  SenseRad=off  SenseAzim=off  SenseDist=off  SenseInc=off  SenseXDot=on  SenseYDot=on  SenseZDot=on  SenseXYZDot=off  SenseRadDot=off  SenseAzimDot=off  SenseDistDot=off  SenseIncDot=off  SenseXDDot=off  SenseYDDot=off  SenseZDDot=off  SenseXYZDDot=off  SenseRadDDot=off  SenseAzimDDot=off  SenseDistDDot=off  SenseIncDDot=off
  Weld Joint : sm_lib/Joints/Weld Joint  JointMode=Normal  CompositeWrenchDir=FollowerOnBase  CompositeWrenchFrame=BaseFrame  SenseConstraintForce=off  SenseConstraintTorque=off  SenseTotalForce=off  SenseTotalTorque=off
  Torso Reference : PMIOPort  Side=Left
  Ground Reference : PMIOPort  Port=2  Side=Left
  Torso Sensing : Outport
  y : Outport  Port=2
  wires:
  PS-Simulink Converter11/1 -> Bus Creator3/2, y/1  "y"
  PS-Simulink Converter/1 -> Bus Creator/1  "wx"
  PS-Simulink Converter2/1 -> Bus Creator/2  "wy"
  PS-Simulink Converter3/1 -> Bus Creator/3  "wz"
  PS-Simulink Converter4/1 -> Bus Creator/4  "x"
  PS-Simulink Converter6/1 -> -z0/1
  PS-Simulink Converter7/1 -> Bus Creator/6  "vx"
  PS-Simulink Converter8/1 -> Bus Creator/7  "vy"
  PS-Simulink Converter9/1 -> Bus Creator/8  "vz"
  -z0/1 -> Bus Creator/5  "dz"
  PS-Simulink Converter10/1 -> Bus Creator1/3  "qz"
  Bus Creator1/1 -> Bus Creator2/1
  PS-Simulink Converter5/1 -> Bus Creator1/2  "qy"
  PS-Simulink Converter1/1 -> Bus Creator1/1  "qx"
  Bus Creator2/1 -> Bus Creator3/1, Torso Sensing/1
  Bus Creator/1 -> Bus Creator2/2
  Bus Creator3/1 -> Scope/1
  connections:
  PS-Simulink Converter6/LConn1 -- Torso Info/RConn7
  PS-Simulink Converter7/LConn1 -- Torso Info/RConn8
  PS-Simulink Converter8/LConn1 -- Torso Info/RConn9
  PS-Simulink Converter9/LConn1 -- Torso Info/RConn10
  Torso Info/RConn1 -- Torso Reference/RConn1 -- Bushing Joint/LConn1
  PS-Simulink Converter/LConn1 -- Torso Info/RConn2
  PS-Simulink Converter4/LConn1 -- Torso Info/RConn5
  PS-Simulink Converter3/LConn1 -- Torso Info/RConn4
  PS-Simulink Converter2/LConn1 -- Torso Info/RConn3
  Bushing Joint/RConn4 -- PS-Simulink Converter10/LConn1
  PS-Simulink Converter5/LConn1 -- Bushing Joint/RConn3
  PS-Simulink Converter1/LConn1 -- Bushing Joint/RConn2
  Align Axes/LConn1 -- Torso Info/LConn1 -- Ground Reference/RConn1
  Torso Info/RConn6 -- PS-Simulink Converter11/LConn1
  Align Axes/RConn1 -- Bushing Joint/RConn1

== system HumanoidModel_ResidualRL/Joint Control/Left Ankle Pitch Control ==
  Control Input : Inport
  Joint Position : Inport  Port=2
  Joint Velocity : Inport  Port=3
  Add Constant : Bias  Bias=jointLowerLimit + (jointUpperLimit-jointLowerLimit)/2  SaturateOnIntegerOverflow=off
  Damping : Gain  Gain=jointDamping
  Degrees to Radians : simulink_extras/Transformations/Degrees to Radians
  Gain : Gain  Gain=(jointUpperLimit-jointLowerLimit)/2
  Stiffness : Gain  Gain=jointStiffness
  Sum1 : Sum  Inputs=|+-
  Sum2 : Sum  Inputs=|+-
  Torque Saturate : Saturate  UpperLimit=jointTorqueLimit  LowerLimit=-jointTorqueLimit  ZeroCross=off
  Torque : Outport
  wires:
  Joint Position/1 -> Sum2/2
  Degrees to Radians/1 -> Sum2/1
  Torque Saturate/1 -> Torque/1
  Sum1/1 -> Torque Saturate/1
  Joint Velocity/1 -> Damping/1
  Sum2/1 -> Stiffness/1
  Control Input/1 -> Gain/1
  Gain/1 -> Add Constant/1
  Add Constant/1 -> Degrees to Radians/1
  Stiffness/1 -> Sum1/1
  Damping/1 -> Sum1/2

== system HumanoidModel_ResidualRL/Joint Control/Left Hip Control ==
  Control Input : Inport
  Joint Position : Inport  Port=2
  Joint Velocity : Inport  Port=3
  Add Constant : Bias  Bias=jointLowerLimit + (jointUpperLimit-jointLowerLimit)/2  SaturateOnIntegerOverflow=off
  Damping : Gain  Gain=jointDamping
  Degrees to Radians : simulink_extras/Transformations/Degrees to Radians
  Gain : Gain  Gain=(jointUpperLimit-jointLowerLimit)/2
  Stiffness : Gain  Gain=jointStiffness
  Sum1 : Sum  Inputs=|+-
  Sum2 : Sum  Inputs=|+-
  Torque Saturate : Saturate  UpperLimit=jointTorqueLimit  LowerLimit=-jointTorqueLimit  ZeroCross=off
  Torque : Outport
  wires:
  Joint Position/1 -> Sum2/2
  Degrees to Radians/1 -> Sum2/1
  Torque Saturate/1 -> Torque/1
  Sum1/1 -> Torque Saturate/1
  Joint Velocity/1 -> Damping/1
  Sum2/1 -> Stiffness/1
  Control Input/1 -> Gain/1
  Gain/1 -> Add Constant/1
  Add Constant/1 -> Degrees to Radians/1
  Stiffness/1 -> Sum1/1
  Damping/1 -> Sum1/2

== system HumanoidModel_ResidualRL/Joint Control/Left Knee Control ==
  Control Input : Inport
  Joint Position : Inport  Port=2
  Joint Velocity : Inport  Port=3
  Add Constant : Bias  Bias=jointLowerLimit + (jointUpperLimit-jointLowerLimit)/2  SaturateOnIntegerOverflow=off
  Damping : Gain  Gain=jointDamping
  Degrees to Radians : simulink_extras/Transformations/Degrees to Radians
  Gain : Gain  Gain=(jointUpperLimit-jointLowerLimit)/2
  Stiffness : Gain  Gain=jointStiffness
  Sum1 : Sum  Inputs=|+-
  Sum2 : Sum  Inputs=|+-
  Torque Saturate : Saturate  UpperLimit=jointTorqueLimit  LowerLimit=-jointTorqueLimit  ZeroCross=off
  Torque : Outport
  wires:
  Joint Position/1 -> Sum2/2
  Degrees to Radians/1 -> Sum2/1
  Torque Saturate/1 -> Torque/1
  Sum1/1 -> Torque Saturate/1
  Joint Velocity/1 -> Damping/1
  Sum2/1 -> Stiffness/1
  Control Input/1 -> Gain/1
  Gain/1 -> Add Constant/1
  Add Constant/1 -> Degrees to Radians/1
  Stiffness/1 -> Sum1/1
  Damping/1 -> Sum1/2

== system HumanoidModel_ResidualRL/Joint Control/Right Ankle Pitch Control ==
  Control Input : Inport
  Joint Position : Inport  Port=2
  Joint Velocity : Inport  Port=3
  Add Constant : Bias  Bias=jointLowerLimit + (jointUpperLimit-jointLowerLimit)/2  SaturateOnIntegerOverflow=off
  Damping : Gain  Gain=jointDamping
  Degrees to Radians : simulink_extras/Transformations/Degrees to Radians
  Gain : Gain  Gain=(jointUpperLimit-jointLowerLimit)/2
  Stiffness : Gain  Gain=jointStiffness
  Sum1 : Sum  Inputs=|+-
  Sum2 : Sum  Inputs=|+-
  Torque Saturate : Saturate  UpperLimit=jointTorqueLimit  LowerLimit=-jointTorqueLimit  ZeroCross=off
  Torque : Outport
  wires:
  Joint Position/1 -> Sum2/2
  Degrees to Radians/1 -> Sum2/1
  Torque Saturate/1 -> Torque/1
  Sum1/1 -> Torque Saturate/1
  Joint Velocity/1 -> Damping/1
  Sum2/1 -> Stiffness/1
  Control Input/1 -> Gain/1
  Gain/1 -> Add Constant/1
  Add Constant/1 -> Degrees to Radians/1
  Stiffness/1 -> Sum1/1
  Damping/1 -> Sum1/2

== system HumanoidModel_ResidualRL/Joint Control/Right Hip Control ==
  Control Input : Inport
  Joint Position : Inport  Port=2
  Joint Velocity : Inport  Port=3
  Add Constant : Bias  Bias=jointLowerLimit + (jointUpperLimit-jointLowerLimit)/2  SaturateOnIntegerOverflow=off
  Damping : Gain  Gain=jointDamping
  Degrees to Radians : simulink_extras/Transformations/Degrees to Radians
  Gain : Gain  Gain=(jointUpperLimit-jointLowerLimit)/2
  Stiffness : Gain  Gain=jointStiffness
  Sum1 : Sum  Inputs=|+-
  Sum2 : Sum  Inputs=|+-
  Torque Saturate : Saturate  UpperLimit=jointTorqueLimit  LowerLimit=-jointTorqueLimit  ZeroCross=off
  Torque : Outport
  wires:
  Joint Position/1 -> Sum2/2
  Degrees to Radians/1 -> Sum2/1
  Torque Saturate/1 -> Torque/1
  Sum1/1 -> Torque Saturate/1
  Joint Velocity/1 -> Damping/1
  Sum2/1 -> Stiffness/1
  Control Input/1 -> Gain/1
  Gain/1 -> Add Constant/1
  Add Constant/1 -> Degrees to Radians/1
  Stiffness/1 -> Sum1/1
  Damping/1 -> Sum1/2

== system HumanoidModel_ResidualRL/Joint Control/Right Hip Sagittal Control ==
  Control Input : Inport
  Joint Position : Inport  Port=2
  Joint Velocity : Inport  Port=3
  Add Constant : Bias  Bias=jointLowerLimit + (jointUpperLimit-jointLowerLimit)/2  SaturateOnIntegerOverflow=off
  Damping : Gain  Gain=jointDamping
  Degrees to Radians : simulink_extras/Transformations/Degrees to Radians
  Gain : Gain  Gain=(jointUpperLimit-jointLowerLimit)/2
  Stiffness : Gain  Gain=jointStiffness
  Sum1 : Sum  Inputs=|+-
  Sum2 : Sum  Inputs=|+-
  Torque Saturate : Saturate  UpperLimit=jointTorqueLimit  LowerLimit=-jointTorqueLimit  ZeroCross=off
  Torque : Outport
  wires:
  Joint Position/1 -> Sum2/2
  Degrees to Radians/1 -> Sum2/1
  Torque Saturate/1 -> Torque/1
  Sum1/1 -> Torque Saturate/1
  Joint Velocity/1 -> Damping/1
  Sum2/1 -> Stiffness/1
  Control Input/1 -> Gain/1
  Gain/1 -> Add Constant/1
  Add Constant/1 -> Degrees to Radians/1
  Stiffness/1 -> Sum1/1
  Damping/1 -> Sum1/2

== system HumanoidModel_ResidualRL/Joint Control/Right Hip Sagittal Control1 ==
  Control Input : Inport
  Joint Position : Inport  Port=2
  Joint Velocity : Inport  Port=3
  Add Constant : Bias  Bias=jointLowerLimit + (jointUpperLimit-jointLowerLimit)/2  SaturateOnIntegerOverflow=off
  Damping : Gain  Gain=jointDamping
  Degrees to Radians : simulink_extras/Transformations/Degrees to Radians
  Gain : Gain  Gain=(jointUpperLimit-jointLowerLimit)/2
  Stiffness : Gain  Gain=jointStiffness
  Sum1 : Sum  Inputs=|+-
  Sum2 : Sum  Inputs=|+-
  Torque Saturate : Saturate  UpperLimit=jointTorqueLimit  LowerLimit=-jointTorqueLimit  ZeroCross=off
  Torque : Outport
  wires:
  Joint Position/1 -> Sum2/2
  Degrees to Radians/1 -> Sum2/1
  Torque Saturate/1 -> Torque/1
  Sum1/1 -> Torque Saturate/1
  Joint Velocity/1 -> Damping/1
  Sum2/1 -> Stiffness/1
  Control Input/1 -> Gain/1
  Gain/1 -> Add Constant/1
  Add Constant/1 -> Degrees to Radians/1
  Stiffness/1 -> Sum1/1
  Damping/1 -> Sum1/2

== system HumanoidModel_ResidualRL/Joint Control/Right Knee Control ==
  Control Input : Inport
  Joint Position : Inport  Port=2
  Joint Velocity : Inport  Port=3
  Add Constant : Bias  Bias=jointLowerLimit + (jointUpperLimit-jointLowerLimit)/2  SaturateOnIntegerOverflow=off
  Damping : Gain  Gain=jointDamping
  Degrees to Radians : simulink_extras/Transformations/Degrees to Radians
  Gain : Gain  Gain=(jointUpperLimit-jointLowerLimit)/2
  Stiffness : Gain  Gain=jointStiffness
  Sum1 : Sum  Inputs=|+-
  Sum2 : Sum  Inputs=|+-
  Torque Saturate : Saturate  UpperLimit=jointTorqueLimit  LowerLimit=-jointTorqueLimit  ZeroCross=off
  Torque : Outport
  wires:
  Joint Position/1 -> Sum2/2
  Degrees to Radians/1 -> Sum2/1
  Torque Saturate/1 -> Torque/1
  Sum1/1 -> Torque Saturate/1
  Joint Velocity/1 -> Damping/1
  Sum2/1 -> Stiffness/1
  Control Input/1 -> Gain/1
  Gain/1 -> Add Constant/1
  Add Constant/1 -> Degrees to Radians/1
  Stiffness/1 -> Sum1/1
  Damping/1 -> Sum1/2

== system HumanoidModel_ResidualRL/Joint Control Arms/Left Shoulder Frontal Control ==
  Control Input : Inport
  Joint Position : Inport  Port=2
  Joint Velocity : Inport  Port=3
  Add Constant : Bias  Bias=jointLowerLimit + (jointUpperLimit-jointLowerLimit)/2  SaturateOnIntegerOverflow=off
  Damping : Gain  Gain=jointDamping
  Degrees to Radians : simulink_extras/Transformations/Degrees to Radians
  Gain : Gain  Gain=(jointUpperLimit-jointLowerLimit)/2
  Stiffness : Gain  Gain=jointStiffness
  Sum1 : Sum  Inputs=|+-
  Sum2 : Sum  Inputs=|+-
  Torque Saturate : Saturate  UpperLimit=jointTorqueLimit  LowerLimit=-jointTorqueLimit  ZeroCross=off
  Torque : Outport
  wires:
  Damping/1 -> Sum1/2
  Stiffness/1 -> Sum1/1
  Add Constant/1 -> Degrees to Radians/1
  Gain/1 -> Add Constant/1
  Control Input/1 -> Gain/1
  Sum2/1 -> Stiffness/1
  Joint Velocity/1 -> Damping/1
  Sum1/1 -> Torque Saturate/1
  Torque Saturate/1 -> Torque/1
  Degrees to Radians/1 -> Sum2/1
  Joint Position/1 -> Sum2/2

== system HumanoidModel_ResidualRL/Joint Control Arms/Right Shoulder Frontal Control ==
  Control Input : Inport
  Joint Position : Inport  Port=2
  Joint Velocity : Inport  Port=3
  Add Constant : Bias  Bias=jointLowerLimit + (jointUpperLimit-jointLowerLimit)/2  SaturateOnIntegerOverflow=off
  Damping : Gain  Gain=jointDamping
  Degrees to Radians : simulink_extras/Transformations/Degrees to Radians
  Gain : Gain  Gain=(jointUpperLimit-jointLowerLimit)/2
  Stiffness : Gain  Gain=jointStiffness
  Sum1 : Sum  Inputs=|+-
  Sum2 : Sum  Inputs=|+-
  Torque Saturate : Saturate  UpperLimit=jointTorqueLimit  LowerLimit=-jointTorqueLimit  ZeroCross=off
  Torque : Outport
  wires:
  Joint Position/1 -> Sum2/2
  Degrees to Radians/1 -> Sum2/1
  Torque Saturate/1 -> Torque/1
  Sum1/1 -> Torque Saturate/1
  Joint Velocity/1 -> Damping/1
  Sum2/1 -> Stiffness/1
  Control Input/1 -> Gain/1
  Gain/1 -> Add Constant/1
  Add Constant/1 -> Degrees to Radians/1
  Stiffness/1 -> Sum1/1
  Damping/1 -> Sum1/2

== system HumanoidModel_ResidualRL/Measurement of PD Torque only/Left Ankle Pitch Control ==
  Control Input : Inport
  Degrees to Radians : simulink_extras/Transformations/Degrees to Radians
  Gain : Gain  Gain=(jointUpperLimit-jointLowerLimit)/2
  Stiffness : Gain  Gain=jointStiffness
  Torque : Outport
  wires:
  Stiffness/1 -> Torque/1
  Degrees to Radians/1 -> Stiffness/1
  Control Input/1 -> Gain/1
  Gain/1 -> Degrees to Radians/1

== system HumanoidModel_ResidualRL/Measurement of PD Torque only/Left Hip Control ==
  Control Input : Inport
  Degrees to Radians : simulink_extras/Transformations/Degrees to Radians
  Gain : Gain  Gain=(jointUpperLimit-jointLowerLimit)/2
  Stiffness : Gain  Gain=jointStiffness
  Torque : Outport
  wires:
  Stiffness/1 -> Torque/1
  Degrees to Radians/1 -> Stiffness/1
  Control Input/1 -> Gain/1
  Gain/1 -> Degrees to Radians/1

== system HumanoidModel_ResidualRL/Measurement of PD Torque only/Left Knee Control ==
  Control Input : Inport
  Degrees to Radians : simulink_extras/Transformations/Degrees to Radians
  Gain : Gain  Gain=(jointUpperLimit-jointLowerLimit)/2
  Stiffness : Gain  Gain=jointStiffness
  Torque : Outport
  wires:
  Stiffness/1 -> Torque/1
  Degrees to Radians/1 -> Stiffness/1
  Control Input/1 -> Gain/1
  Gain/1 -> Degrees to Radians/1

== system HumanoidModel_ResidualRL/Measurement of PD Torque only/Nominal u ==
  Constant : Constant  Value=u_hip_frontal
  Constant1 : Constant  Value=u_knee
  Constant{5..6,10..11} (4 alike) : Constant  Value=0
  Constant2 : Constant  Value=u_ankle_pitch
  Constant3 : Constant  Value=u_hip_sagittal
  Constant4 : Constant  Value=u_hip_sagittal
  Constant7 : Constant  Value=u_knee
  Constant8 : Constant  Value=u_ankle_pitch
  Constant9 : Constant  Value=u_hip_frontal
  Mux : Mux  Inputs=12
  Out1 : Outport
  wires:
  Constant9/1 -> Mux/7  "Left Hip Frontal"
  Constant/1 -> Mux/1  "Right Hip Frontal"
  Constant6/1 -> Mux/6  "Right Ankle Roll"
  Constant8/1 -> Mux/9  "Left Ankle Pitch"
  Constant7/1 -> Mux/8  "Left Knee"
  Constant5/1 -> Mux/5  "Right Hip Transverse"
  Constant3/1 -> Mux/4  "Right Hip Sagittal"
  Constant2/1 -> Mux/3  "Right Ankle Pitch"
  Constant11/1 -> Mux/12  "Left Ankle Roll"
  Constant4/1 -> Mux/10  "Left Hip Sagittal"
  Constant1/1 -> Mux/2  "Right Knee"
  Constant10/1 -> Mux/11  "Left Hip Transverse"
  Mux/1 -> Out1/1

== system HumanoidModel_ResidualRL/Measurement of PD Torque only/Right Ankle Pitch Control ==
  Control Input : Inport
  Degrees to Radians : simulink_extras/Transformations/Degrees to Radians
  Gain : Gain  Gain=(jointUpperLimit-jointLowerLimit)/2
  Stiffness : Gain  Gain=jointStiffness
  Torque : Outport
  wires:
  Stiffness/1 -> Torque/1
  Degrees to Radians/1 -> Stiffness/1
  Control Input/1 -> Gain/1
  Gain/1 -> Degrees to Radians/1

== system HumanoidModel_ResidualRL/Measurement of PD Torque only/Right Hip Control ==
  Control Input : Inport
  Degrees to Radians : simulink_extras/Transformations/Degrees to Radians
  Gain : Gain  Gain=(jointUpperLimit-jointLowerLimit)/2
  Stiffness : Gain  Gain=jointStiffness
  Torque : Outport
  wires:
  Stiffness/1 -> Torque/1
  Degrees to Radians/1 -> Stiffness/1
  Control Input/1 -> Gain/1
  Gain/1 -> Degrees to Radians/1

== system HumanoidModel_ResidualRL/Measurement of PD Torque only/Right Hip Sagittal Control ==
  Control Input : Inport
  Degrees to Radians : simulink_extras/Transformations/Degrees to Radians
  Gain : Gain  Gain=(jointUpperLimit-jointLowerLimit)/2
  Stiffness : Gain  Gain=jointStiffness
  Torque : Outport
  wires:
  Stiffness/1 -> Torque/1
  Degrees to Radians/1 -> Stiffness/1
  Control Input/1 -> Gain/1
  Gain/1 -> Degrees to Radians/1

== system HumanoidModel_ResidualRL/Measurement of PD Torque only/Right Hip Sagittal Control1 ==
  Control Input : Inport
  Degrees to Radians : simulink_extras/Transformations/Degrees to Radians
  Gain : Gain  Gain=(jointUpperLimit-jointLowerLimit)/2
  Stiffness : Gain  Gain=jointStiffness
  Torque : Outport
  wires:
  Stiffness/1 -> Torque/1
  Degrees to Radians/1 -> Stiffness/1
  Control Input/1 -> Gain/1
  Gain/1 -> Degrees to Radians/1

== system HumanoidModel_ResidualRL/Measurement of PD Torque only/Right Knee Control ==
  Control Input : Inport
  Degrees to Radians : simulink_extras/Transformations/Degrees to Radians
  Gain : Gain  Gain=(jointUpperLimit-jointLowerLimit)/2
  Stiffness : Gain  Gain=jointStiffness
  Torque : Outport
  wires:
  Stiffness/1 -> Torque/1
  Degrees to Radians/1 -> Stiffness/1
  Control Input/1 -> Gain/1
  Gain/1 -> Degrees to Radians/1

== system HumanoidModel_ResidualRL/Humanoid Robot/Arms/Left Arm ==
  Torque Input : Inport
  Bus Creator : BusCreator  Inputs=2
  Demux : Demux  Outputs=2
  Elbow Joint : Subsystem
  Hand : sm_lib/Body Elements/File Solid  ExtGeomFileName=sm_humanoid_walker_hand.stp  UnitType=FromFile  ExtGeomFileUnits=m  StepReaderType=HEX  ExportConvexHullGeometry=off  InertiaType=CalculateFromGeometry  BasedOnType=Density  Density=handDensity  DensityUnits=kg/m^3  Mass=0  MassUnits=kg  CenterOfMass=[0, 0, 0]  CenterOfMassUnits=m  MomentsOfInertia=[0, 0, 0]  MomentsOfInertiaUnits=kg*m^2  ProductsOfInertia=[0, 0, 0]  ProductsOfInertiaUnits=kg*m^2  GraphicType=FromGeometry  MarkerShape=Sphere  MarkerSize=10  GraphicVisPropType=SimpleVisualProperties  GraphicDiffuseColor=[0.3, 0.3, 0.3]  GraphicOpacity=1  GraphicSpecularColor=[0.5 0.5 0.5 1.0]  GraphicAmbientColor=[0.15 0.15 0.15 1.0]  GraphicEmissiveColor=[0.0 0.0 0.0 1.0]  GraphicShininess=75  DoExposeReferenceFrame=on  SerializedFrames=<Frames/>
  Lower Arm : sm_lib/Body Elements/File Solid  ExtGeomFileName=sm_humanoid_walker_lower_arm.stp  UnitType=FromFile  ExtGeomFileUnits=m  StepReaderType=HEX  ExportConvexHullGeometry=off  InertiaType=CalculateFromGeometry  BasedOnType=Density  Density=lowerArmDensity  DensityUnits=kg/m^3  Mass=0  MassUnits=kg  CenterOfMass=[0, 0, 0]  CenterOfMassUnits=m  MomentsOfInertia=[0, 0, 0]  MomentsOfInertiaUnits=kg*m^2  ProductsOfInertia=[0, 0, 0]  ProductsOfInertiaUnits=kg*m^2  GraphicType=FromGeometry  MarkerShape=Sphere  MarkerSize=10  GraphicVisPropType=SimpleVisualProperties  GraphicDiffuseColor=[1, 1, 1]  GraphicOpacity=1  GraphicSpecularColor=[0.5 0.5 0.5 1.0]  GraphicAmbientColor=[0.15 0.15 0.15 1.0]  GraphicEmissiveColor=[0.0 0.0 0.0 1.0]  GraphicShininess=75  DoExposeReferenceFrame=on  SerializedFrames=<Frames/>
  Shoulder Frontal Joint : Subsystem
  Shoulder Sagittal Joint : Subsystem
  Shoulder Swivel : sm_lib/Body Elements/File Solid  ExtGeomFileName=sm_humanoid_walker_shoulder_swivel.stp  UnitType=FromFile  ExtGeomFileUnits=m  StepReaderType=HEX  ExportConvexHullGeometry=off  InertiaType=CalculateFromGeometry  BasedOnType=Density  Density=shoulderDensity  DensityUnits=kg/m^3  Mass=0  MassUnits=kg  CenterOfMass=[0, 0, 0]  CenterOfMassUnits=m  MomentsOfInertia=[0, 0, 0]  MomentsOfInertiaUnits=kg*m^2  ProductsOfInertia=[0, 0, 0]  ProductsOfInertiaUnits=kg*m^2  GraphicType=FromGeometry  MarkerShape=Sphere  MarkerSize=10  GraphicVisPropType=SimpleVisualProperties  GraphicDiffuseColor=[0.3, 0.3, 0.3]  GraphicOpacity=1  GraphicSpecularColor=[0.5 0.5 0.5 1.0]  GraphicAmbientColor=[0.15 0.15 0.15 1.0]  GraphicEmissiveColor=[0.0 0.0 0.0 1.0]  GraphicShininess=75  DoExposeReferenceFrame=on  SerializedFrames=<Frames/>
  Upper Arm : sm_lib/Body Elements/File Solid  ExtGeomFileName=sm_humanoid_walker_upper_arm.stp  UnitType=FromFile  ExtGeomFileUnits=m  StepReaderType=HEX  ExportConvexHullGeometry=off  InertiaType=CalculateFromGeometry  BasedOnType=Density  Density=upperArmDensity  DensityUnits=kg/m^3  Mass=0  MassUnits=kg  CenterOfMass=[0, 0, 0]  CenterOfMassUnits=m  MomentsOfInertia=[0, 0, 0]  MomentsOfInertiaUnits=kg*m^2  ProductsOfInertia=[0, 0, 0]  ProductsOfInertiaUnits=kg*m^2  GraphicType=FromGeometry  MarkerShape=Sphere  MarkerSize=10  GraphicVisPropType=SimpleVisualProperties  GraphicDiffuseColor=[1, 1, 1]  GraphicOpacity=1  GraphicSpecularColor=[0.5 0.5 0.5 1.0]  GraphicAmbientColor=[0.15 0.15 0.15 1.0]  GraphicEmissiveColor=[0.0 0.0 0.0 1.0]  GraphicShininess=75  DoExposeReferenceFrame=on  SerializedFrames=<Frames/>
  Wrist Joint : Subsystem
  Left Shoulder : PMIOPort  Side=Left
  Sensing : Outport
  wires:
  Torque Input/1 -> Demux/1
  Bus Creator/1 -> Sensing/1
  Demux/1 -> Shoulder Frontal Joint/1(Torque)
  Shoulder Frontal Joint/1(Sensing) -> Bus Creator/1
  Demux/2 -> Shoulder Sagittal Joint/1(Torque)
  Shoulder Sagittal Joint/1(Sensing) -> Bus Creator/2
  connections:
  Hand/RConn1 -- Wrist Joint/RConn1
  Wrist Joint/LConn1 -- Lower Arm/RConn1 -- Elbow Joint/RConn1
  Shoulder Frontal Joint/LConn1 -- Left Shoulder/RConn1
  Shoulder Swivel/RConn1 -- Shoulder Sagittal Joint/LConn1 -- Shoulder Frontal Joint/RConn1
  Upper Arm/RConn1 -- Elbow Joint/LConn1 -- Shoulder Sagittal Joint/RConn1
